simulink model "Tinkercad"  (R2022a)
settings: Solver=FixedStepAuto  StartTime=0.0  StopTime=10.0  RelTol=1e-3
settings Model: Creator=Arman  LastModifiedBy=parsa
settings OptimizationCC: DefaultParameterBehavior=Inlined  UseDivisionForNetSlopeComputation=on  GainParamInheritBuiltInType=on  UseFloatMulNetSlope=on  InlineInvariantSignals=on  PassReuseOutputArgsAs=Individual arguments  ZeroExternalMemoryAtStartup=off  ZeroInternalMemoryAtStartup=off  NoFixptDivByZeroProtection=on  EfficientFloat2IntCast=on  LifeSpan=1  OptimizeBlockOrder=speed  DifferentSizesBufferReuse=on  EfficientTunableParamExpr=on
settings DebuggingCC: ParameterTunabilityLossMsg=error
settings HardwareCC: ProdLongLongMode=on
settings SFSimCC: MATLABDynamicMemAlloc=off
settings RTWCC: SystemTargetFile=ert.tlc  TemplateMakefile=ert_default_tmf
settings CodeAppCC: ForceParamTrailComments=on  IgnoreCustomStorageClasses=off  OperatorAnnotations=on  SimulinkDataObjDesc=on  SFDataObjDesc=on  CustomSymbolStrGlobalVar=rt$N$M  CustomSymbolStrType=$N$M  CustomSymbolStrFcn=$N$M$F  CustomSymbolStrMacro=$N$M  InsertBlockDesc=on
settings ERTTargetCC: TargetLangStandard=C99 (ISO)  GenerateSampleERTMain=on  IncludeMdlTerminateFcn=off  CombineSignalStateStructs=on  SupportComplex=off  SupportContinuousTime=on  SupportNonInlinedSFcns=on  InlinedParameterPlacement=NonHierarchical  ERTCustomFileTemplate=example_file_process.tlc  ERTFilePackagingFormat=CompactWithDataFile

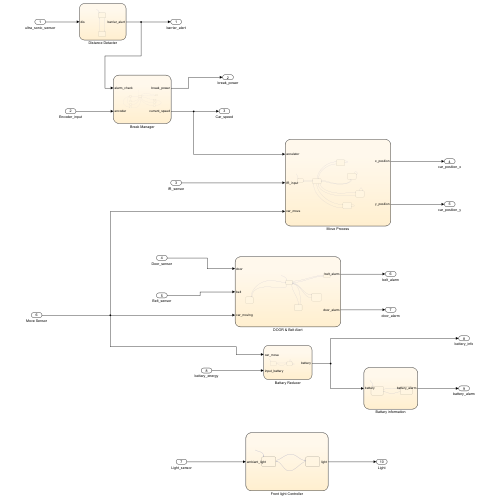
[thumbnail: Simulink's stored preview of the top-level diagram]
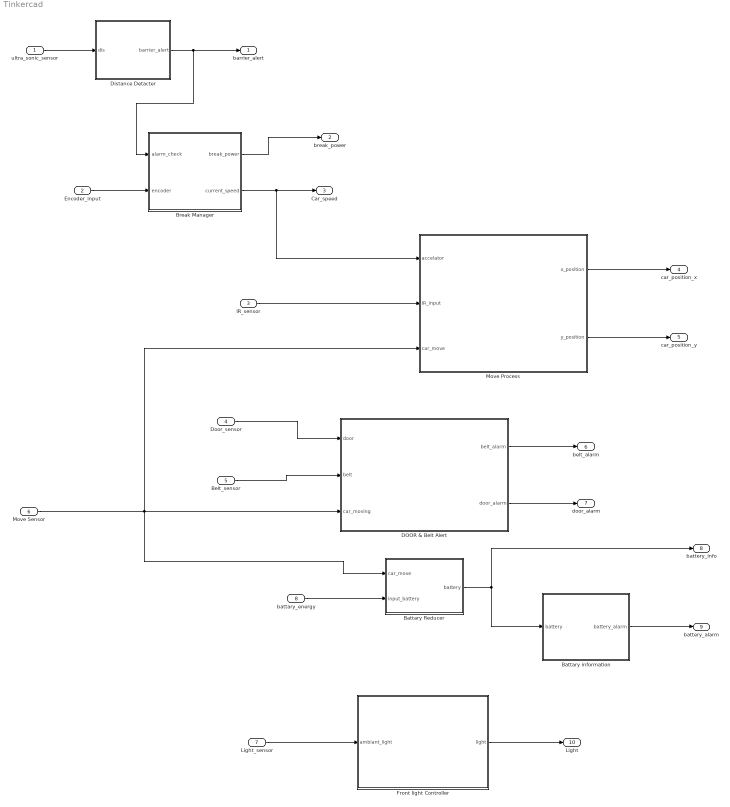
== system Tinkercad ==
  ultra_sonic_sensor : Inport
  Encoder_input : Inport  Port=2
  IR_sensor : Inport  Port=3
  Door_sensor : Inport  Port=4
  Belt_sensor : Inport  Port=5
  Move Sensor : Inport  Port=6
  Light_sensor : Inport  Port=7
  battary_energy : Inport  Port=8
  Battary Reducer : Stateflow chart  TreatAsAtomicUnit=on
  Battary information : Stateflow chart  TreatAsAtomicUnit=on
  Break Manager : Stateflow chart  TreatAsAtomicUnit=on
      settings: PortSchema="{\"entries\":[{\"content\":{\"sides\":[{\"content\":{\"connectorIds\":[\"In2\",\"In1\"]},\"type\":\"ConnectorPlacement.EquallySpacedRectSide\",\"uuid\":\"2ee3b5d0-505a-4a26-bfe9-7ec1ca943a7a\"},{\"content\":{\"connectorIds\":[\"Out1\",\"Out2\"],\"side\":\"RIGHT\"},\"type\":\"ConnectorPlacement.EquallySpacedRectSide\",\"uuid\":\"c507a312-3aa6-42ad-943d-24377cbf621f\"},{\"content\":{\"connectorIds\":[],\"side\":\"TOP\"},\"type\":\"ConnectorPlacement.EquallySpacedRectSide\",\"uuid\":\"4f690229-4f51-4b44-9769-e2a1a70a1308\"}]},\"type\":\"ConnectorPlacement.EquallySpacedConnector\",\"uuid\":\"51d36195-2b79-4537-b363-bdd1e932f082\"}],\"packageUris\":[\"http://schema.mathworks.com/mf0/Connector/R2020b\"],\"version\":\"1.0\"}"
  DOOR & Belt Alert : Stateflow chart  TreatAsAtomicUnit=on
      settings: PortSchema="{\"entries\":[{\"content\":{\"sides\":[{\"content\":{\"connectorIds\":[\"In1\",\"In3\",\"In2\"]},\"type\":\"ConnectorPlacement.EquallySpacedRectSide\",\"uuid\":\"ef0a918c-b3da-4393-92bd-86778b9479e8\"},{\"content\":{\"connectorIds\":[\"Out1\",\"Out2\"],\"side\":\"RIGHT\"},\"type\":\"ConnectorPlacement.EquallySpacedRectSide\",\"uuid\":\"5393d4fd-b470-4389-b50f-325c6a759493\"},{\"content\":{\"connectorIds\":[],\"side\":\"TOP\"},\"type\":\"ConnectorPlacement.EquallySpacedRectSide\",\"uuid\":\"e7dd1106-fbbb-4601-86dd-49977af21262\"}]},\"type\":\"ConnectorPlacement.EquallySpacedConnector\",\"uuid\":\"c5f3d552-669d-4b32-9fa9-d2033a64bbde\"}],\"packageUris\":[\"http://schema.mathworks.com/mf0/Connector/R2020b\"],\"version\":\"1.0\"}"
  Distance Detacter : Stateflow chart  TreatAsAtomicUnit=on
  Front light Controller : Stateflow chart  TreatAsAtomicUnit=on
  Move Process : Stateflow chart  TreatAsAtomicUnit=on
  barrier_alert : Outport
  break_power : Outport  Port=2
  Car_speed : Outport  Port=3
  car_position_x : Outport  Port=4
  car_position_y : Outport  Port=5
  belt_alarm : Outport  Port=6
  door_alarm : Outport  Port=7
  battery_info : Outport  Port=8
  battery_alarm : Outport  Port=9
  Light : Outport  Port=10
  wires:
  Break Manager/1(break_power) -> break_power/1
  Distance Detacter/1(barrier_alert) -> Break Manager/2(alarm_check), barrier_alert/1
  Move Process/2(y_position) -> car_position_y/1
  Battary Reducer/1(battery) -> battery_info/1, Battary information/1(battery)
  Front light Controller/1(light) -> Light/1
  Door_sensor/1 -> DOOR & Belt Alert/1(door)
  Move Process/1(x_position) -> car_position_x/1
  ultra_sonic_sensor/1 -> Distance Detacter/1(dis)
  Move Sensor/1 -> Move Process/3(car_move), Battary Reducer/1(car_move), DOOR & Belt Alert/2(car_moving)
  DOOR & Belt Alert/1(belt_alarm) -> belt_alarm/1
  Belt_sensor/1 -> DOOR & Belt Alert/3(belt)
  Encoder_input/1 -> Break Manager/1(encoder)
  Battary information/1(battery_alarm) -> battery_alarm/1
  IR_sensor/1 -> Move Process/2(IR_input)
  DOOR & Belt Alert/2(door_alarm) -> door_alarm/1
  Light_sensor/1 -> Front light Controller/1(ambiant_light)
  battary_energy/1 -> Battary Reducer/2(input_battery)
  Break Manager/2(current_speed) -> Car_speed/1, Move Process/1(accelator)

== stateflow chart Tinkercad/DOOR & Belt Alert ==
  state d_alarm_off
  state idel
  state d_alarm_on
  state b_alarm_on
  state b_alarm_off
  (default) -> idel : {door_alarm = 0; belt_alarm = 0;}
  idel -> d_alarm_off [order 4] : [door == 0 && door_alarm ==1]{door_alarm=0;}
  d_alarm_off -> idel
  b_alarm_on -> idel
  idel -> d_alarm_on [order 3] : [door == 1 && door_alarm == 0]{door_alarm = 1}
  b_alarm_off -> idel
  d_alarm_on -> idel
  idel -> b_alarm_on [order 1] : [car_moving == 1 && belt == 0 && belt_alarm == 0]{belt_alarm = 1;}
  idel -> b_alarm_off [order 2] : [(belt == 1 && belt_alarm == 1) || (car_moving == 0 && belt_alarm == 1)]{belt_alarm = 0;}
  data: door input; car_moving input; belt input; belt_alarm output; door_alarm output

== stateflow chart Tinkercad/Front light Controller ==
  state light_off
  state Light_on
  (default) -> light_off : {light = 0;}
  light_off -> Light_on : [ambiant_light < 0]{light = 1}
  Light_on -> light_off : [ambiant_light >= 0]{light = 0}
  data: ambiant_light input; light output

== stateflow chart Tinkercad/Battary information ==
  state not_low_battery
  state low_battery
  (default) -> not_low_battery : {battery_alarm = 0;}
  not_low_battery -> low_battery : [battery <= 20]{battery_alarm = 1;}
  low_battery -> not_low_battery : [battery > 20]{battery_alarm =0;}
  data: battery input; battery_alarm output

== stateflow chart Tinkercad/Battary Reducer ==
  state No_battery_reduse
  state Battery_reduser
  (default) -> No_battery_reduse : {battery = input_battery;}
  Battery_reduser -> Battery_reduser [order 2] : [timer <= 5000 && battery > 0 ]{timer = timer + 1;}
  No_battery_reduse -> Battery_reduser : [car_move ==1]{timer = 0;}
  Battery_reduser -> No_battery_reduse [order 1] : [car_move == 0]
  Battery_reduser -> Battery_reduser [order 3] : [timer > 5000]{battery = battery - 1;timer = 0;}
  data: car_move input; input_battery input; timer local; battery output

== stateflow chart Tinkercad/Distance Detacter ==
  state safe
  state alarm
  (default) -> safe : {barrier_alert = 0}
  alarm -> safe : [dis > 160]{barrier_alert = 0}
  safe -> alarm : [dis <= 160]{barrier_alert = 1}
  data: dis input; barrier_alert output

== stateflow chart Tinkercad/Break Manager ==
  state speed_cal
  state alarm_on
  state idel
  state Change_speed
  state low_brak
  state speed_rise
  state mid_brak
  state speed_fall
  state hard_brak
  (default) -> idel : {current_speed = 0; static_speed = 5; c_speed = 0;
      | last_encode=0;break_power = 0;}
  idel -> speed_cal [order 1] : [after(3,sec) && (encoder - last_encode <= 6.5 && encoder - last_encode >= - 6.5 )]
  speed_cal -> idel : {current_speed = (static_speed*c_speed) - (break_power*c_speed);
      | break_power = 0;}
  idel -> alarm_on [order 3] : [alarm_check== 1]
  alarm_on -> hard_brak [order 3] : [ encoder > 20]
      | {break_power = 4;}
  alarm_on -> mid_brak [order 2] : [encoder > 10 && encoder<20]
      | {brak_power = 3;}
  idel -> Change_speed [order 2] : [after(3,sec) && (encoder - last_encode > 6.5 || encoder - last_encode < -6.5)]
  alarm_on -> low_brak [order 1] : [encoder < 10]
      | {brak_power = 2;}
  low_brak -> idel : {current_speed = (static_speed*c_speed) - (brak_power*c_speed)}
  hard_brak -> idel : {current_speed = (static_speed*c_speed) - (brak_power*c_speed)}
  mid_brak -> idel : {current_speed = (static_speed*c_speed) - (brak_power*c_speed)}
  speed_fall -> idel : {
      | last_encode = encoder;
      | c_speed = c_speed -1;
      | }
  speed_rise -> idel : {
      | last_encode = encoder;
      | c_speed = c_speed +1;
      | }
  Change_speed -> speed_rise [order 1] : [encoder - last_encode > 6.5]
  Change_speed -> speed_fall [order 2] : [encoder - last_encode < -6.5]
  data: encoder input; alarm_check input; break_power output; c_speed local; last_encode local; static_speed local; current_speed output

== stateflow chart Tinkercad/Move Process ==
  state straight_up
    % the car must go up
  state straight_down
    % the car must go down
  state Stop_car
  state Start_move
    %car start moving
  state straight_left
    % the car must go left
  state straight_right
    % the car must go right
  straight_up -> straight_up [order 2] : [IR_input == 17]{y_position = y_position + accelator;}
  Start_move -> straight_up [order 2] : [IR_input == 17]{y_position = y_position + accelator;}
  straight_up -> Start_move [order 1] : [IR_input ~= 17]
  straight_down -> straight_down [order 2] : [IR_input == 25]{y_position = y_position - accelator;}
  (default) -> Stop_car : {x_position=0;y_position=0;}
  Start_move -> straight_down [order 3] : [IR_input == 25]{y_position = y_position - accelator;}
  straight_down -> Start_move [order 1] : [IR_input ~= 25]
  Stop_car -> Start_move : [car_move == 1]
  Start_move -> Stop_car [order 1] : [car_move==0]
  straight_right -> Start_move [order 1] : [IR_input ~= 22]
  Start_move -> straight_right [order 5] : [IR_input == 22]{x_position = x_position + accelator;}
  straight_left -> Start_move [order 1] : [IR_input ~= 20]
  Start_move -> straight_left [order 4] : [IR_input == 20]{x_position = x_position - accelator;}
  straight_left -> straight_left [order 2] : [IR_input == 20]{x_position = x_position - accelator;}
  straight_right -> straight_right [order 2] : [IR_input == 22]{x_position = x_position + accelator;}
  data: accelator input; IR_input input; car_move input; x_position output; y_position output
